simulink model "Grua_MC_R2_Ciclo_Completo_SFC"  (R2025b)
settings: Solver=ode23t  StartTime=0.0  StopTime=640  MaxStep=T_s  RelTol=1e-4
InitFcn:
  | addpath(fileparts(get_param(bdroot,'FileName')),'-begin');
  | run(fullfile(fileparts(get_param(bdroot,'FileName')),'definir_buses_variadores.m'));
  | run(fullfile(fileparts(get_param(bdroot,'FileName')),'parametros_ganancias_cascada_29072026.m'));
  | run(fullfile(fileparts(get_param(bdroot,'FileName')),'configurar_modelo_final_hmi.m'));
  | run(fullfile(fileparts(get_param(bdroot,'FileName')),'configurar_parametros_variadores.m'));
  | Pvis.Ts_viz=.04;Pvis.enable=true;Pvis.keepFigureOnTerminate=true;Pvis.hmi.fastDiagnostic=false;
undefined symbols (not defined in the file or in its folder): b_cx, b_cy, b_hb, b_hEb, b_heq, b_t, b_tb, b_teq, b_tw, b_wu, g, H_c, HMI, i_h, i_t, J_heq, J_teq, K_cy, K_tw, k_wu, L_h0, l_hi, M_c_profile, M_s, M_t, MC_FF, nLevels0, omega_hmRATED, r_hd, r_td, slotBlock, T_hbMax, T_hEbMax, T_hmMax, T_s, T_s1, T_tbMax, T_tmMax, tau_hm, tau_tm, traj_duration, traj_x_start, traj_x_target, v_hmaxLoaded, v_hmaxUnloaded, x_tmax, x_tmin, Y_c0, Y_t0, Zbase
libraries: simulink x1, aerolibanimutils x1
(part 3 of 4)

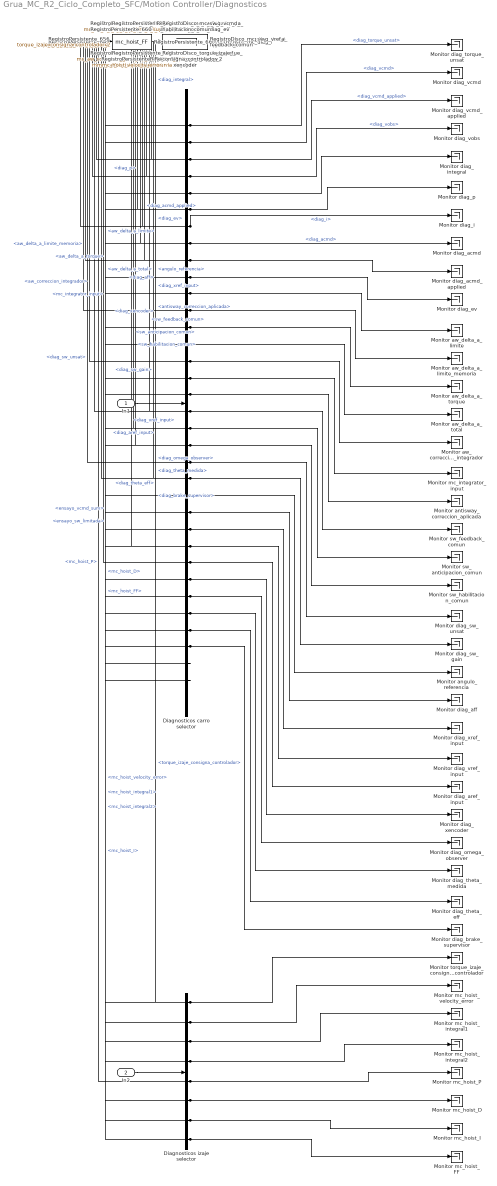
== system Grua_MC_R2_Ciclo_Completo_SFC/Motion Controller/Diagnosticos ==
  In1 : Inport
  In2 : Inport  Port=2
  Diagnosticos carro selector : BusSelector  OutputSignals=diag_torque_unsat,diag_vcmd,diag_vcmd_applied,diag_vobs,diag_integral,diag_p,diag_i,diag_acmd,diag_acmd_applied,diag_ev,aw_delta_a_limite,aw_delta_a_limite_memoria,aw_delta_a_torque,aw_delta_a_total,aw_correccion_integrador,mc_integrator_input,antisway_correccion_aplicada,sw_feedback_comun,sw_anticipacion_comun,sw_habilitacion_comun,diag_sw_unsat,diag_sw_gain,angulo_referencia,diag_aff,diag_xref_input,diag_vref_input,diag_aref_input,diag_xencoder,diag_omega_observer,diag_theta_medida,diag_theta_eff,diag_brake_supervisor,ensayo_vcmd_sum,ensayo_sw_limitada
  Diagnosticos izaje selector : BusSelector  OutputSignals=torque_izaje_consigna_controlador,mc_hoist_velocity_error,mc_hoist_integral1,mc_hoist_integral2,mc_hoist_P,mc_hoist_D,mc_hoist_I,mc_hoist_FF
  Monitor angulo_referencia : Terminator
  Monitor antisway_correccion_aplicada : Terminator
  Monitor aw_correccion_integrador : Terminator
  Monitor aw_delta_a_limite : Terminator
  Monitor aw_delta_a_limite_memoria : Terminator
  Monitor aw_delta_a_torque : Terminator
  Monitor aw_delta_a_total : Terminator
  Monitor diag_acmd : Terminator
  Monitor diag_acmd_applied : Terminator
  Monitor diag_aff : Terminator
  Monitor diag_aref_input : Terminator
  Monitor diag_brake_supervisor : Terminator
  Monitor diag_ev : Terminator
  Monitor diag_i : Terminator
  Monitor diag_integral : Terminator
  Monitor diag_omega_observer : Terminator
  Monitor diag_p : Terminator
  Monitor diag_sw_gain : Terminator
  Monitor diag_sw_unsat : Terminator
  Monitor diag_theta_eff : Terminator
  Monitor diag_theta_medida : Terminator
  Monitor diag_torque_unsat : Terminator
  Monitor diag_vcmd : Terminator
  Monitor diag_vcmd_applied : Terminator
  Monitor diag_vobs : Terminator
  Monitor diag_vref_input : Terminator
  Monitor diag_xencoder : Terminator
  Monitor diag_xref_input : Terminator
  Monitor mc_hoist_D : Terminator
  Monitor mc_hoist_FF : Terminator
  Monitor mc_hoist_I : Terminator
  Monitor mc_hoist_P : Terminator
  Monitor mc_hoist_integral1 : Terminator
  Monitor mc_hoist_integral2 : Terminator
  Monitor mc_hoist_velocity_error : Terminator
  Monitor mc_integrator_input : Terminator
  Monitor sw_anticipacion_comun : Terminator
  Monitor sw_feedback_comun : Terminator
  Monitor sw_habilitacion_comun : Terminator
  Monitor torque_izaje_consigna_controlador : Terminator
  RegistroDisco_angulo_referencia : Terminator
  RegistroDisco_mc_antisway_correccion_aplicada : Terminator
  RegistroDisco_mc_diag_acmd : Terminator
  RegistroDisco_mc_diag_acmd_applied : Terminator
  RegistroDisco_mc_diag_aff : Terminator
  RegistroDisco_mc_diag_aref_input : Terminator
  RegistroDisco_mc_diag_brake_supervisor : Terminator
  RegistroDisco_mc_diag_ev : Terminator
  RegistroDisco_mc_diag_i : Terminator
  RegistroDisco_mc_diag_integral : Terminator
  RegistroDisco_mc_diag_omega_observer : Terminator
  RegistroDisco_mc_diag_p : Terminator
  RegistroDisco_mc_diag_sw_gain : Terminator
  RegistroDisco_mc_diag_theta_eff : Terminator
  RegistroDisco_mc_diag_theta_medida : Terminator
  RegistroDisco_mc_diag_torque_unsat : Terminator
  RegistroDisco_mc_diag_vcmd : Terminator
  RegistroDisco_mc_diag_vcmd_applied : Terminator
  RegistroDisco_mc_diag_vobs : Terminator
  RegistroDisco_mc_diag_vref_input : Terminator
  RegistroDisco_mc_diag_xencoder : Terminator
  RegistroDisco_mc_diag_xref_input : Terminator
  RegistroDisco_mc_sw_anticipacion_comun : Terminator
  RegistroDisco_mc_sw_feedback_comun : Terminator
  RegistroDisco_mc_sw_habilitacion_comun : Terminator
  RegistroDisco_torque_izaje_consigna_controlador_2 : Terminator
  RegistroPersistente_622 : ToWorkspace  VariableName=mc_diag_torque_unsat  SaveFormat=Timeseries  SampleTime=-1
      settings: Decimation=10
  RegistroPersistente_623 : ToWorkspace  VariableName=mc_diag_vcmd  SaveFormat=Timeseries  SampleTime=-1
      settings: Decimation=10
  RegistroPersistente_624 : ToWorkspace  VariableName=mc_diag_vcmd_applied  SaveFormat=Timeseries  SampleTime=-1
      settings: Decimation=10
  RegistroPersistente_625 : ToWorkspace  VariableName=mc_diag_vobs  SaveFormat=Timeseries  SampleTime=-1
      settings: Decimation=10
  RegistroPersistente_626 : ToWorkspace  VariableName=mc_diag_integral  SaveFormat=Timeseries  SampleTime=-1
      settings: Decimation=10
  RegistroPersistente_627 : ToWorkspace  VariableName=mc_diag_p  SaveFormat=Timeseries  SampleTime=-1
      settings: Decimation=10
  RegistroPersistente_628 : ToWorkspace  VariableName=mc_diag_i  SaveFormat=Timeseries  SampleTime=-1
      settings: Decimation=10
  RegistroPersistente_629 : ToWorkspace  VariableName=mc_diag_acmd  SaveFormat=Timeseries  SampleTime=-1
      settings: Decimation=10
  RegistroPersistente_630 : ToWorkspace  VariableName=mc_diag_acmd_applied  SaveFormat=Timeseries  SampleTime=-1
      settings: Decimation=10
  RegistroPersistente_631 : ToWorkspace  VariableName=mc_diag_ev  SaveFormat=Timeseries  SampleTime=-1
      settings: Decimation=10
  RegistroPersistente_632 : ToWorkspace  VariableName=mc_aw_delta_a_limite  SaveFormat=Timeseries  SampleTime=-1
      settings: Decimation=10
  RegistroPersistente_633 : ToWorkspace  VariableName=mc_aw_delta_a_limite_memoria  SaveFormat=Timeseries  SampleTime=-1
      settings: Decimation=10
  RegistroPersistente_634 : ToWorkspace  VariableName=mc_aw_delta_a_torque  SaveFormat=Timeseries  SampleTime=-1
      settings: Decimation=10
  RegistroPersistente_635 : ToWorkspace  VariableName=mc_aw_delta_a_total  SaveFormat=Timeseries  SampleTime=-1
      settings: Decimation=10
  RegistroPersistente_636 : ToWorkspace  VariableName=mc_aw_correccion_integrador  SaveFormat=Timeseries  SampleTime=-1
      settings: Decimation=10
  RegistroPersistente_637 : ToWorkspace  VariableName=mc_mc_integrator_input  SaveFormat=Timeseries  SampleTime=-1
      settings: Decimation=10
  RegistroPersistente_638 : ToWorkspace  VariableName=mc_antisway_correccion_aplicada  SaveFormat=Timeseries  SampleTime=-1
      settings: Decimation=10
  RegistroPersistente_639 : ToWorkspace  VariableName=mc_sw_feedback_comun  SaveFormat=Timeseries  SampleTime=-1
      settings: Decimation=10
  RegistroPersistente_640 : ToWorkspace  VariableName=mc_sw_anticipacion_comun  SaveFormat=Timeseries  SampleTime=-1
      settings: Decimation=10
  RegistroPersistente_641 : ToWorkspace  VariableName=mc_sw_habilitacion_comun  SaveFormat=Timeseries  SampleTime=-1
      settings: Decimation=10
  RegistroPersistente_642 : ToWorkspace  VariableName=antisway_calculada  SaveFormat=Timeseries  SampleTime=-1
      settings: Decimation=10
  RegistroPersistente_643 : ToWorkspace  VariableName=mc_diag_sw_gain  SaveFormat=Timeseries  SampleTime=-1
      settings: Decimation=10
  RegistroPersistente_644 : ToWorkspace  VariableName=angulo_referencia  SaveFormat=Timeseries  SampleTime=-1
      settings: Decimation=10
  RegistroPersistente_645 : ToWorkspace  VariableName=mc_diag_aff  SaveFormat=Timeseries  SampleTime=-1
      settings: Decimation=10
  RegistroPersistente_646 : ToWorkspace  VariableName=mc_diag_xref_input  SaveFormat=Timeseries  SampleTime=-1
      settings: Decimation=10
  RegistroPersistente_647 : ToWorkspace  VariableName=mc_diag_vref_input  SaveFormat=Timeseries  SampleTime=-1
      settings: Decimation=10
  RegistroPersistente_648 : ToWorkspace  VariableName=mc_diag_aref_input  SaveFormat=Timeseries  SampleTime=-1
      settings: Decimation=10
  RegistroPersistente_649 : ToWorkspace  VariableName=mc_diag_xencoder  SaveFormat=Timeseries  SampleTime=-1
      settings: Decimation=10
  RegistroPersistente_650 : ToWorkspace  VariableName=mc_diag_omega_observer  SaveFormat=Timeseries  SampleTime=-1
      settings: Decimation=10
  RegistroPersistente_651 : ToWorkspace  VariableName=mc_diag_theta_medida  SaveFormat=Timeseries  SampleTime=-1
      settings: Decimation=10
  RegistroPersistente_652 : ToWorkspace  VariableName=mc_diag_theta_eff  SaveFormat=Timeseries  SampleTime=-1
      settings: Decimation=10
  RegistroPersistente_653 : ToWorkspace  VariableName=mc_diag_brake_supervisor  SaveFormat=Timeseries  SampleTime=-1
      settings: Decimation=10
  RegistroPersistente_654 : ToWorkspace  VariableName=v_cmd  SaveFormat=Timeseries  SampleTime=-1
      settings: Decimation=10
  RegistroPersistente_655 : ToWorkspace  VariableName=antisway_limitada  SaveFormat=Timeseries  SampleTime=-1
      settings: Decimation=10
  RegistroPersistente_656 : ToWorkspace  VariableName=torque_izaje_consigna_controlador_2  SaveFormat=Timeseries  SampleTime=-1
      settings: Decimation=10
  RegistroPersistente_657 : ToWorkspace  VariableName=mc_hoist_velocity_error  SaveFormat=Timeseries  SampleTime=-1
      settings: Decimation=10
  RegistroPersistente_658 : ToWorkspace  VariableName=mc_hoist_integral1  SaveFormat=Timeseries  SampleTime=-1
      settings: Decimation=10
  RegistroPersistente_659 : ToWorkspace  VariableName=mc_hoist_integral2  SaveFormat=Timeseries  SampleTime=-1
      settings: Decimation=10
  RegistroPersistente_660 : ToWorkspace  VariableName=mc_hoist_P  SaveFormat=Timeseries  SampleTime=-1
      settings: Decimation=10
  RegistroPersistente_661 : ToWorkspace  VariableName=mc_hoist_D  SaveFormat=Timeseries  SampleTime=-1
      settings: Decimation=10
  RegistroPersistente_662 : ToWorkspace  VariableName=mc_hoist_I  SaveFormat=Timeseries  SampleTime=-1
      settings: Decimation=10
  RegistroPersistente_663 : ToWorkspace  VariableName=mc_hoist_FF  SaveFormat=Timeseries  SampleTime=-1
      settings: Decimation=10
  wires:
  Diagnosticos izaje selector/6 -> Monitor mc_hoist_D/1, RegistroPersistente_661/1  "<mc_hoist_D>"
  Diagnosticos carro selector/27 -> Monitor diag_aref_input/1, RegistroPersistente_648/1, RegistroDisco_mc_diag_aref_input/1  "<diag_aref_input>"
  In1/1 -> Diagnosticos carro selector/1
  Diagnosticos carro selector/22 -> Monitor diag_sw_gain/1, RegistroPersistente_643/1, RegistroDisco_mc_diag_sw_gain/1  "<diag_sw_gain>"
  Diagnosticos izaje selector/5 -> Monitor mc_hoist_P/1, RegistroPersistente_660/1  "<mc_hoist_P>"
  Diagnosticos carro selector/3 -> Monitor diag_vcmd_applied/1, RegistroPersistente_624/1, RegistroDisco_mc_diag_vcmd_applied/1  "<diag_vcmd_applied>"
  Diagnosticos carro selector/18 -> Monitor sw_feedback_comun/1, RegistroPersistente_639/1, RegistroDisco_mc_sw_feedback_comun/1  "<sw_feedback_comun>"
  Diagnosticos carro selector/4 -> Monitor diag_vobs/1, RegistroPersistente_625/1, RegistroDisco_mc_diag_vobs/1  "<diag_vobs>"
  Diagnosticos carro selector/15 -> Monitor aw_correccion_integrador/1, RegistroPersistente_636/1  "<aw_correccion_integrador>"
  In2/1 -> Diagnosticos izaje selector/1
  Diagnosticos carro selector/21 -> Monitor diag_sw_unsat/1, RegistroPersistente_642/1  "<diag_sw_unsat>"
  Diagnosticos carro selector/9 -> Monitor diag_acmd_applied/1, RegistroPersistente_630/1, RegistroDisco_mc_diag_acmd_applied/1  "<diag_acmd_applied>"
  Diagnosticos carro selector/12 -> Monitor aw_delta_a_limite_memoria/1, RegistroPersistente_633/1  "<aw_delta_a_limite_memoria>"
  Diagnosticos carro selector/7 -> Monitor diag_i/1, RegistroPersistente_628/1, RegistroDisco_mc_diag_i/1  "<diag_i>"
  Diagnosticos carro selector/8 -> Monitor diag_acmd/1, RegistroPersistente_629/1, RegistroDisco_mc_diag_acmd/1  "<diag_acmd>"
  Diagnosticos carro selector/6 -> Monitor diag_p/1, RegistroPersistente_627/1, RegistroDisco_mc_diag_p/1  "<diag_p>"
  Diagnosticos carro selector/20 -> Monitor sw_habilitacion_comun/1, RegistroPersistente_641/1, RegistroDisco_mc_sw_habilitacion_comun/1  "<sw_habilitacion_comun>"
  Diagnosticos carro selector/19 -> Monitor sw_anticipacion_comun/1, RegistroPersistente_640/1, RegistroDisco_mc_sw_anticipacion_comun/1  "<sw_anticipacion_comun>"
  Diagnosticos carro selector/26 -> Monitor diag_vref_input/1, RegistroPersistente_647/1, RegistroDisco_mc_diag_vref_input/1  "<diag_vref_input>"
  Diagnosticos carro selector/11 -> Monitor aw_delta_a_limite/1, RegistroPersistente_632/1  "<aw_delta_a_limite>"
  Diagnosticos carro selector/32 -> Monitor diag_brake_supervisor/1, RegistroPersistente_653/1, RegistroDisco_mc_diag_brake_supervisor/1  "<diag_brake_supervisor>"
  Diagnosticos carro selector/13 -> Monitor aw_delta_a_torque/1, RegistroPersistente_634/1  "<aw_delta_a_torque>"
  Diagnosticos carro selector/2 -> Monitor diag_vcmd/1, RegistroPersistente_623/1, RegistroDisco_mc_diag_vcmd/1  "<diag_vcmd>"
  Diagnosticos carro selector/17 -> Monitor antisway_correccion_aplicada/1, RegistroPersistente_638/1, RegistroDisco_mc_antisway_correccion_aplicada/1  "<antisway_correccion_aplicada>"
  Diagnosticos izaje selector/1 -> Monitor torque_izaje_consigna_controlador/1, RegistroPersistente_656/1, RegistroDisco_torque_izaje_consigna_controlador_2/1  "<torque_izaje_consigna_controlador>"
  Diagnosticos carro selector/10 -> Monitor diag_ev/1, RegistroPersistente_631/1, RegistroDisco_mc_diag_ev/1  "<diag_ev>"
  Diagnosticos carro selector/1 -> Monitor diag_torque_unsat/1, RegistroPersistente_622/1, RegistroDisco_mc_diag_torque_unsat/1  "<diag_torque_unsat>"
  Diagnosticos carro selector/5 -> Monitor diag_integral/1, RegistroPersistente_626/1, RegistroDisco_mc_diag_integral/1  "<diag_integral>"
  Diagnosticos carro selector/16 -> Monitor mc_integrator_input/1, RegistroPersistente_637/1  "<mc_integrator_input>"
  Diagnosticos izaje selector/4 -> Monitor mc_hoist_integral2/1, RegistroPersistente_659/1  "<mc_hoist_integral2>"
  Diagnosticos izaje selector/2 -> Monitor mc_hoist_velocity_error/1, RegistroPersistente_657/1  "<mc_hoist_velocity_error>"
  Diagnosticos izaje selector/3 -> Monitor mc_hoist_integral1/1, RegistroPersistente_658/1  "<mc_hoist_integral1>"
  Diagnosticos carro selector/14 -> Monitor aw_delta_a_total/1, RegistroPersistente_635/1  "<aw_delta_a_total>"
  Diagnosticos carro selector/28 -> Monitor diag_xencoder/1, RegistroPersistente_649/1, RegistroDisco_mc_diag_xencoder/1  "<diag_xencoder>"
  Diagnosticos carro selector/24 -> Monitor diag_aff/1, RegistroPersistente_645/1, RegistroDisco_mc_diag_aff/1  "<diag_aff>"
  Diagnosticos carro selector/23 -> Monitor angulo_referencia/1, RegistroPersistente_644/1, RegistroDisco_angulo_referencia/1  "<angulo_referencia>"
  Diagnosticos carro selector/30 -> Monitor diag_theta_medida/1, RegistroPersistente_651/1, RegistroDisco_mc_diag_theta_medida/1  "<diag_theta_medida>"
  Diagnosticos carro selector/31 -> Monitor diag_theta_eff/1, RegistroPersistente_652/1, RegistroDisco_mc_diag_theta_eff/1  "<diag_theta_eff>"
  Diagnosticos carro selector/29 -> Monitor diag_omega_observer/1, RegistroPersistente_650/1, RegistroDisco_mc_diag_omega_observer/1  "<diag_omega_observer>"
  Diagnosticos carro selector/25 -> Monitor diag_xref_input/1, RegistroPersistente_646/1, RegistroDisco_mc_diag_xref_input/1  "<diag_xref_input>"
  Diagnosticos izaje selector/8 -> Monitor mc_hoist_FF/1, RegistroPersistente_663/1  "<mc_hoist_FF>"
  Diagnosticos izaje selector/7 -> Monitor mc_hoist_I/1, RegistroPersistente_662/1  "<mc_hoist_I>"
  Diagnosticos carro selector/33 -> RegistroPersistente_654/1  "<ensayo_vcmd_sum>"
  Diagnosticos carro selector/34 -> RegistroPersistente_655/1  "<ensayo_sw_limitada>"

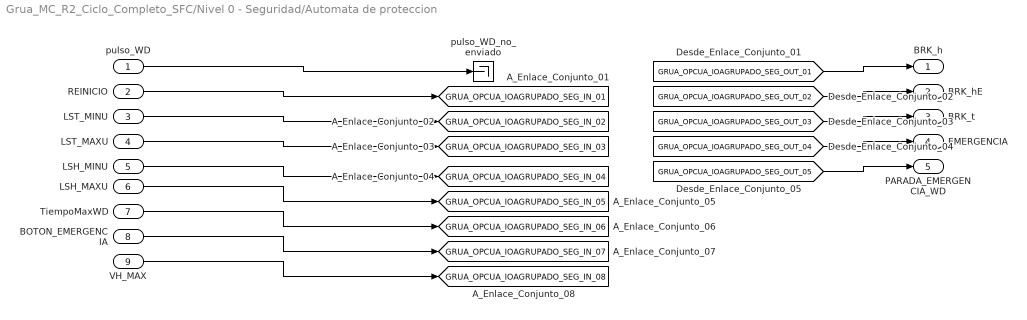
== system Grua_MC_R2_Ciclo_Completo_SFC/Nivel 0 - Seguridad/Automata de proteccion ==
  pulso_WD : Inport
  REINICIO : Inport  Port=2
  LST_MINU : Inport  Port=3
  LST_MAXU : Inport  Port=4
  LSH_MINU : Inport  Port=5
  LSH_MAXU : Inport  Port=6
  TiempoMaxWD : Inport  Port=7
  BOTON_EMERGENCIA : Inport  Port=8
  VH_MAX : Inport  Port=9
  pulso_WD_no_enviado : Terminator
  BRK_h : Outport
  BRK_hE : Outport  Port=2
  BRK_t : Outport  Port=3
  EMERGENCIA : Outport  Port=4
  PARADA_EMERGENCIA_WD : Outport  Port=5
  tag scope: GRUA_OPCUA_IOAGRUPADO_SEG_IN_01=global, GRUA_OPCUA_IOAGRUPADO_SEG_IN_02=global, GRUA_OPCUA_IOAGRUPADO_SEG_IN_03=global, GRUA_OPCUA_IOAGRUPADO_SEG_IN_04=global, GRUA_OPCUA_IOAGRUPADO_SEG_IN_05=global, GRUA_OPCUA_IOAGRUPADO_SEG_IN_06=global, GRUA_OPCUA_IOAGRUPADO_SEG_IN_07=global, GRUA_OPCUA_IOAGRUPADO_SEG_IN_08=global
  wires:
  [GRUA_OPCUA_IOAGRUPADO_SEG_OUT_05] -> PARADA_EMERGENCIA_WD/1
  [GRUA_OPCUA_IOAGRUPADO_SEG_OUT_04] -> EMERGENCIA/1
  [GRUA_OPCUA_IOAGRUPADO_SEG_OUT_03] -> BRK_t/1
  [GRUA_OPCUA_IOAGRUPADO_SEG_OUT_02] -> BRK_hE/1
  [GRUA_OPCUA_IOAGRUPADO_SEG_OUT_01] -> BRK_h/1
  VH_MAX/1 -> [GRUA_OPCUA_IOAGRUPADO_SEG_IN_08]
  BOTON_EMERGENCIA/1 -> [GRUA_OPCUA_IOAGRUPADO_SEG_IN_07]
  TiempoMaxWD/1 -> [GRUA_OPCUA_IOAGRUPADO_SEG_IN_06]
  LSH_MAXU/1 -> [GRUA_OPCUA_IOAGRUPADO_SEG_IN_05]
  LSH_MINU/1 -> [GRUA_OPCUA_IOAGRUPADO_SEG_IN_04]
  LST_MAXU/1 -> [GRUA_OPCUA_IOAGRUPADO_SEG_IN_03]
  LST_MINU/1 -> [GRUA_OPCUA_IOAGRUPADO_SEG_IN_02]
  REINICIO/1 -> [GRUA_OPCUA_IOAGRUPADO_SEG_IN_01]
  pulso_WD/1 -> pulso_WD_no_enviado/1

== system Grua_MC_R2_Ciclo_Completo_SFC/Planta/Calculo longitud l ==
  x_l : Inport
  y_l : Inport  Port=2
  v_lx : Inport  Port=3
  v_ly : Inport  Port=4
  x_t : Inport  Port=5
  v_t : Inport  Port=6
  Constant : Constant  Value=Y_t0
  Divide : Product  Inputs=*/
  Product : Product
  Product1 : Product
  Sqrt : Sqrt
  Square : Math  Operator=square
  Square1 : Math  Operator=square
  Sum : Sum  Inputs=|+-
  Sum1 : Sum  Inputs=|+-
  Sum2 : Sum
  Sum3 : Sum  Inputs=|+-
  Sum4 : Sum  Inputs=+-
  l : Outport
  dl : Outport  Port=2
  wires:
  Sqrt/1 -> Divide/2, l/1  "l"
  x_l/1 -> Sum/1
  x_t/1 -> Sum/2
  Sum/1 -> Product/1, Square/1
  Constant/1 -> Sum1/1
  y_l/1 -> Sum1/2
  Sum1/1 -> Product1/1, Square1/1
  Square1/1 -> Sum2/2
  Square/1 -> Sum2/1
  Sum2/1 -> Sqrt/1
  v_lx/1 -> Sum3/1
  v_t/1 -> Sum3/2
  Sum3/1 -> Product/2
  v_ly/1 -> Product1/2
  Product1/1 -> Sum4/2
  Product/1 -> Sum4/1
  Sum4/1 -> Divide/1
  Divide/1 -> dl/1  "dl"

== system Grua_MC_R2_Ciclo_Completo_SFC/Planta/Subsistema carga ==
  x_t : Inport
  F_w : Inport  Port=2
  M_c : Inport  Port=3
  y_c0(x_l,t) : Inport  Port=4
  TLK : Inport  Port=5
  Calculo Angulo De Balanceo : Subsystem
  Calculo Fuerza De Contacto : Subsystem
  Calculo Longitud Inferior : Subsystem
  Calculo Masa Total de Carga : Subsystem
  Derivative : Derivative
  Dinamica Movimiento Carga : Subsystem
  RegistroDisco_masa_fisica_suspendida : Terminator
  RegistroDisco_v_izaje_fisica : Terminator
  RegistroDisco_y_carga_fisica : Terminator
  RegistroPersistente_830 : ToWorkspace  VariableName=masa_fisica_suspendida  SaveFormat=Timeseries  SampleTime=-1
      settings: Decimation=10
  RegistroPersistente_838 : ToWorkspace  VariableName=y_carga_fisica  SaveFormat=Timeseries  SampleTime=-1
      settings: Decimation=10
  RegistroPersistente_840 : ToWorkspace  VariableName=v_izaje_fisica  SaveFormat=Timeseries  SampleTime=-1
      settings: Decimation=10
  x_l : Outport
  y_l : Outport  Port=2
  v_lx : Outport  Port=3
  v_ly : Outport  Port=4
  theta_l : Outport  Port=5
  omega_l : Outport  Port=6
  F_cy : Outport  Port=7
  wires:
  Calculo Fuerza De Contacto/2(F_cy) -> F_cy/1, Dinamica Movimiento Carga/3(F_cy)
  Dinamica Movimiento Carga/4(v_ly) -> v_ly/1, Calculo Fuerza De Contacto/3(v_ly), RegistroPersistente_840/1, RegistroDisco_v_izaje_fisica/1
  x_t/1 -> Calculo Angulo De Balanceo/3(x_t)
  Dinamica Movimiento Carga/2(y_l) -> y_l/1, Calculo Angulo De Balanceo/2(y_l), Calculo Fuerza De Contacto/1(y_l), RegistroPersistente_838/1, RegistroDisco_y_carga_fisica/1
  Calculo Angulo De Balanceo/1(theta_l) -> Dinamica Movimiento Carga/5(theta_l), Derivative/1, theta_l/1
  y_c0(x_l,t)/1 -> Calculo Fuerza De Contacto/5(y_c0(x_l,t))
  Calculo Fuerza De Contacto/1(F_cx) -> Dinamica Movimiento Carga/2(F_cx)
  Dinamica Movimiento Carga/1(x_l) -> x_l/1, Calculo Angulo De Balanceo/1(x_l)
  Dinamica Movimiento Carga/3(v_lx) -> v_lx/1, Calculo Fuerza De Contacto/2(v_lx)
  Calculo Longitud Inferior/1(h_c) -> Calculo Fuerza De Contacto/4(h_c)
  F_w/1 -> Dinamica Movimiento Carga/4(F_hw)
  M_c/1 -> Calculo Masa Total de Carga/2(M_c)
  TLK/1 -> Calculo Longitud Inferior/1(TLK), Calculo Masa Total de Carga/1(TLK)
  Derivative/1 -> omega_l/1
  Calculo Masa Total de Carga/1(m_l) -> Dinamica Movimiento Carga/1(m_l), RegistroPersistente_830/1, RegistroDisco_masa_fisica_suspendida/1

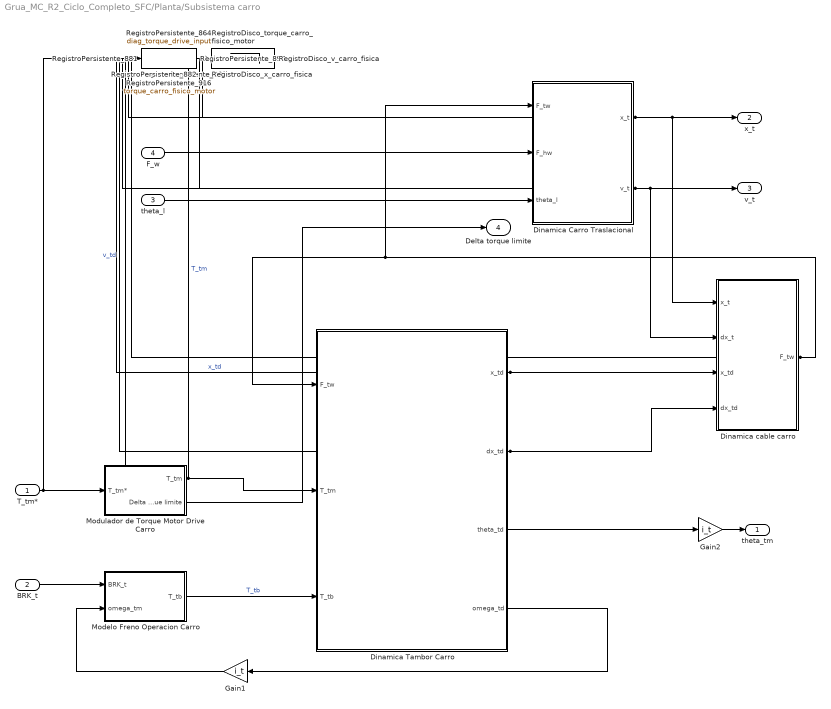
== system Grua_MC_R2_Ciclo_Completo_SFC/Planta/Subsistema carro ==
  T_tm* : Inport
  BRK_t : Inport  Port=2
  theta_l : Inport  Port=3
  F_w : Inport  Port=4
  Dinamica Carro Traslacional : Subsystem
  Dinamica Tambor Carro : Subsystem
  Dinamica cable carro : Subsystem
  Gain1 : Gain  Gain=i_t
  Gain2 : Gain  Gain=i_t
  Modelo Freno Operacion Carro : Subsystem
  Modulador de Torque Motor Drive Carro : Subsystem
  RegistroDisco_torque_carro_fisico_motor : Terminator
  RegistroDisco_v_carro_fisica : Terminator
  RegistroDisco_x_carro_fisica : Terminator
  RegistroPersistente_864 : ToWorkspace  VariableName=diag_torque_drive_input  SaveFormat=Timeseries  SampleTime=-1
      settings: Decimation=10
  RegistroPersistente_868 : ToWorkspace  VariableName=x_carro_fisica  SaveFormat=Timeseries  SampleTime=-1
      settings: Decimation=10
  RegistroPersistente_869 : ToWorkspace  VariableName=v_carro_fisica  SaveFormat=Timeseries  SampleTime=-1
      settings: Decimation=10
  RegistroPersistente_881 : ToWorkspace  VariableName=x_td  SaveFormat=Timeseries  SampleTime=-1
      settings: Decimation=10
  RegistroPersistente_882 : ToWorkspace  VariableName=v_td  SaveFormat=Timeseries  SampleTime=-1
      settings: Decimation=10
  RegistroPersistente_897 : ToWorkspace  VariableName=diag_traction  SaveFormat=Timeseries  SampleTime=-1
      settings: Decimation=10
  RegistroPersistente_916 : ToWorkspace  VariableName=torque_carro_fisico_motor  SaveFormat=Timeseries  SampleTime=-1
      settings: Decimation=10
  theta_tm : Outport
  x_t : Outport  Port=2
  v_t : Outport  Port=3
  Delta torque limite : Outport  Port=4
  wires:
  Dinamica cable carro/1(F_tw) -> Dinamica Carro Traslacional/1(F_tw), Dinamica Tambor Carro/1(F_tw), RegistroPersistente_897/1
  Gain1/1 -> Modelo Freno Operacion Carro/2(omega_tm)
  F_w/1 -> Dinamica Carro Traslacional/2(F_hw)
  Dinamica Carro Traslacional/1(x_t) -> x_t/1, Dinamica cable carro/1(x_t), RegistroPersistente_868/1, RegistroDisco_x_carro_fisica/1
  Modulador de Torque Motor Drive Carro/1(T_tm) -> Dinamica Tambor Carro/2(T_tm), RegistroPersistente_916/1, RegistroDisco_torque_carro_fisico_motor/1  "T_tm"
  Dinamica Tambor Carro/4(omega_td) -> Gain1/1
  Dinamica Carro Traslacional/2(v_t) -> v_t/1, Dinamica cable carro/2(dx_t), RegistroPersistente_869/1, RegistroDisco_v_carro_fisica/1
  Dinamica Tambor Carro/2(dx_td) -> Dinamica cable carro/4(dx_td), RegistroPersistente_882/1  "v_td"
  Dinamica Tambor Carro/1(x_td) -> Dinamica cable carro/3(x_td), RegistroPersistente_881/1  "x_td"
  Modelo Freno Operacion Carro/1(T_tb) -> Dinamica Tambor Carro/3(T_tb)  "T_tb"
  BRK_t/1 -> Modelo Freno Operacion Carro/1(BRK_t)
  Dinamica Tambor Carro/3(theta_td) -> Gain2/1
  T_tm*/1 -> Modulador de Torque Motor Drive Carro/1(T_tm*), RegistroPersistente_864/1
  theta_l/1 -> Dinamica Carro Traslacional/3(theta_l)
  Gain2/1 -> theta_tm/1
  Modulador de Torque Motor Drive Carro/2(Delta torque limite) -> Delta torque limite/1

== system Grua_MC_R2_Ciclo_Completo_SFC/Planta/Subsistema izaje ==
  F_hw : Inport
  BRK_hE : Inport  Port=2
  T_hm* : Inport  Port=3
  BRK_h : Inport  Port=4
  l : Inport  Port=5
  dl : Inport  Port=6
  Calculo longitud l_h : Subsystem
  Dinamica Tambor Izaje : Subsystem
  Dinamica cable Izaje : Subsystem
  Gain : Gain  Gain=i_h
  Gain1 : Gain  Gain=i_h
  Modelo Freno Emergencia de Izaje(Eje lento) : Subsystem
  Modelo Freno Operacion de Izaje(Eje Rapido) : Subsystem
  Modulador de Torque Motor Drive Izaje : Subsystem
  RegistroDisco_torque_izaje_fisico_motor : Terminator
  RegistroPersistente_934 : ToWorkspace  VariableName=l_h  SaveFormat=Timeseries  SampleTime=-1
      settings: Decimation=10
  RegistroPersistente_992 : ToWorkspace  VariableName=torque_izaje_fisico_motor  SaveFormat=Timeseries  SampleTime=-1
      settings: Decimation=10
  theta_hd : Outport
  theta_hm : Outport  Port=2
  F_w : Outport  Port=3
  omega_hd : Outport  Port=4
  wires:
  Calculo longitud l_h/1(l_h) -> Dinamica cable Izaje/2(l_h), RegistroPersistente_934/1  "l_h"
  Calculo longitud l_h/2(dl_h) -> Dinamica cable Izaje/4(dl_h)
  F_hw/1 -> Dinamica Tambor Izaje/3(F_hw)
  Modelo Freno Emergencia de Izaje(Eje lento)/1(T_hEb) -> Dinamica Tambor Izaje/1(T_hEb)
  Dinamica Tambor Izaje/1(theta_hd) -> Gain1/1, theta_hd/1
  BRK_h/1 -> Modelo Freno Operacion de Izaje(Eje Rapido)/1(BRK_h)
  Modelo Freno Operacion de Izaje(Eje Rapido)/1(T_hb) -> Dinamica Tambor Izaje/4(T_hb)
  Gain/1 -> Modulador de Torque Motor Drive Izaje/2(omega_hm), Modelo Freno Operacion de Izaje(Eje Rapido)/2(omega_hm)
  BRK_hE/1 -> Modelo Freno Emergencia de Izaje(Eje lento)/2(BRK_hE)
  T_hm*/1 -> Modulador de Torque Motor Drive Izaje/1(T_hm*)
  l/1 -> Dinamica cable Izaje/1(l)
  Dinamica cable Izaje/1(F_hw) -> F_w/1  "F_w"
  dl/1 -> Dinamica cable Izaje/3(dl)
  Modulador de Torque Motor Drive Izaje/1(T_hm) -> Dinamica Tambor Izaje/2(T_hm), RegistroPersistente_992/1, RegistroDisco_torque_izaje_fisico_motor/1
  Gain1/1 -> theta_hm/1
  Dinamica Tambor Izaje/2(omega_hd) -> Gain/1, Modelo Freno Emergencia de Izaje(Eje lento)/1(omega_hd), Calculo longitud l_h/1(omega_hd), omega_hd/1

== system Grua_MC_R2_Ciclo_Completo_SFC/SENSORES/Finales de carrera operacion carro ==
  x_t : Inport
  Constant : Constant  Value=x_tmax
  Constant1 : Constant  Value=x_tmin
  Constant2 : Constant  Value=x_tmax+0.50
  Constant3 : Constant  Value=x_tmin-0.50
  Relational Operator{1..4} (4 alike) : RelationalOperator  OutDataTypeStr=boolean  RndMeth=Simplest  InputSameDT=off
  x_tLSmax : Outport
  x_tLSmin : Outport  Port=2
  x_tLSEmax : Outport  Port=3
  x_tLSEmin : Outport  Port=4
  wires:
  Relational Operator4/1 -> x_tLSmax/1
  Constant/1 -> Relational Operator4/2
  Constant1/1 -> Relational Operator1/1
  x_t/1 -> Relational Operator3/2, Relational Operator2/1, Relational Operator1/2, Relational Operator4/1
  Relational Operator1/1 -> x_tLSmin/1
  Relational Operator3/1 -> x_tLSEmin/1
  Relational Operator2/1 -> x_tLSEmax/1
  Constant2/1 -> Relational Operator2/2
  Constant3/1 -> Relational Operator3/1

== system Grua_MC_R2_Ciclo_Completo_SFC/SENSORES/Sensor de Sobrevelocidad>115% ==
  v_h : Inport
  TLK : Inport  Port=2
  Abs : Abs  SaturateOnIntegerOverflow=off
  Constant : Constant  Value=v_hmaxLoaded
  Constant1 : Constant  Value=v_hmaxUnloaded
  Gain : Gain  Gain=1.15
  Relational Operator : RelationalOperator  OutDataTypeStr=boolean  RndMeth=Simplest  InputSameDT=off
  Switch : Switch  Criteria=u2 > Threshold  SaturateOnIntegerOverflow=off  InputSameDT=off
  Sobrevelocidad : Outport
  wires:
  Switch/1 -> Gain/1  "v_hlim"
  Constant/1 -> Switch/1
  TLK/1 -> Switch/2
  Constant1/1 -> Switch/3
  v_h/1 -> Abs/1
  Relational Operator/1 -> Sobrevelocidad/1
  Gain/1 -> Relational Operator/2
  Abs/1 -> Relational Operator/1

== system Grua_MC_R2_Ciclo_Completo_SFC/SENSORES/Subsystem1 ==
  theta_l : Inport
  omega_l : Inport  Port=2
  sensor angulo vertical : Gain
  sensor de velocidad angular : Gain
  theta_l_sensor : Outport
  omega_l_sensor : Outport  Port=2
  wires:
  sensor angulo vertical/1 -> theta_l_sensor/1
  sensor de velocidad angular/1 -> omega_l_sensor/1
  omega_l/1 -> sensor de velocidad angular/1
  theta_l/1 -> sensor angulo vertical/1

== system Grua_MC_R2_Ciclo_Completo_SFC/Planta/Subsistema carga/Calculo Angulo De Balanceo ==
  x_l : Inport
  y_l : Inport  Port=2
  x_t : Inport  Port=3
  Atan : Trigonometry  Operator=atan2
  Constant : Constant  Value=Y_t0
  RegistroPersistente_802 : ToWorkspace  VariableName=x_l  SaveFormat=Timeseries  SampleTime=-1
      settings: Decimation=10
  RegistroPersistente_803 : ToWorkspace  VariableName=y_l  SaveFormat=Timeseries  SampleTime=-1
      settings: Decimation=10
  RegistroPersistente_804 : ToWorkspace  VariableName=x_t  SaveFormat=Timeseries  SampleTime=-1
      settings: Decimation=10
  Sum : Sum  Inputs=|+-
  Sum1 : Sum  Inputs=|+-
  theta_l : Outport
  wires:
  x_l/1 -> Sum/1, RegistroPersistente_802/1  "x_l"
  x_t/1 -> Sum/2, RegistroPersistente_804/1  "x_t"
  Constant/1 -> Sum1/1
  y_l/1 -> Sum1/2, RegistroPersistente_803/1  "y_l"
  Sum/1 -> Atan/1
  Sum1/1 -> Atan/2
  Atan/1 -> theta_l/1

== system Grua_MC_R2_Ciclo_Completo_SFC/Planta/Subsistema carga/Calculo Fuerza De Contacto ==
  y_l : Inport
  v_lx : Inport  Port=2
  v_ly : Inport  Port=3
  h_c : Inport  Port=4
  y_c0(x_l,t) : Inport  Port=5
  Constant1 : Constant  Value=0
  Gain : Gain  Gain=-b_cx
  Gain1 : Gain  Gain=K_cy
  Gain2 : Gain  Gain=-b_cy
  Limite fuerza contacto : Saturate  UpperLimit=2e6  LowerLimit=0
  RegistroPersistente_821 : ToWorkspace  VariableName=sumFcx  SaveFormat=Timeseries  SampleTime=-1
      settings: Decimation=10
  RegistroPersistente_823 : ToWorkspace  VariableName=registro_823  SaveFormat=Timeseries  SampleTime=-1
      settings: Decimation=10
  Sum : Sum  Inputs=++-
  Sum1 : Sum  Inputs=|++
  Switch : Switch  SaturateOnIntegerOverflow=off  InputSameDT=off
  Switch1 : Switch  SaturateOnIntegerOverflow=off  InputSameDT=off
  F_cx : Outport
  F_cy : Outport  Port=2
  wires:
  Switch/1 -> F_cx/1, RegistroPersistente_823/1
  Constant1/1 -> Switch1/3, Switch/3
  Gain/1 -> Switch/1
  h_c/1 -> Sum/2
  y_c0(x_l,t)/1 -> Sum/1
  y_l/1 -> Sum/3
  Sum/1 -> Gain1/1, Switch1/2, Switch/2, RegistroPersistente_821/1  "sumFcx"
  v_lx/1 -> Gain/1
  Gain1/1 -> Sum1/1
  Gain2/1 -> Sum1/2
  v_ly/1 -> Gain2/1
  Sum1/1 -> Switch1/1
  Switch1/1 -> Limite fuerza contacto/1
  Limite fuerza contacto/1 -> F_cy/1

== system Grua_MC_R2_Ciclo_Completo_SFC/Planta/Subsistema carga/Calculo Longitud Inferior ==
  TLK : Inport
  Constant : Constant  Value=H_c
  Constant1 : Constant  Value=0
  Switch : Switch  Criteria=u2 > Threshold  SaturateOnIntegerOverflow=off  InputSameDT=off
  h_c : Outport
  wires:
  TLK/1 -> Switch/2
  Switch/1 -> h_c/1
  Constant1/1 -> Switch/3
  Constant/1 -> Switch/1

== system Grua_MC_R2_Ciclo_Completo_SFC/Planta/Subsistema carga/Calculo Masa Total de Carga ==
  TLK : Inport
  M_c : Inport  Port=2
  Constant : Constant  Value=M_s
  Sum : Sum  Inputs=|++
  Switch : Switch  Criteria=u2 > Threshold  SaturateOnIntegerOverflow=off  InputSameDT=off
  m_l : Outport
  wires:
  TLK/1 -> Switch/2
  M_c/1 -> Sum/2
  Switch/1 -> m_l/1
  Constant/1 -> Sum/1, Switch/3
  Sum/1 -> Switch/1

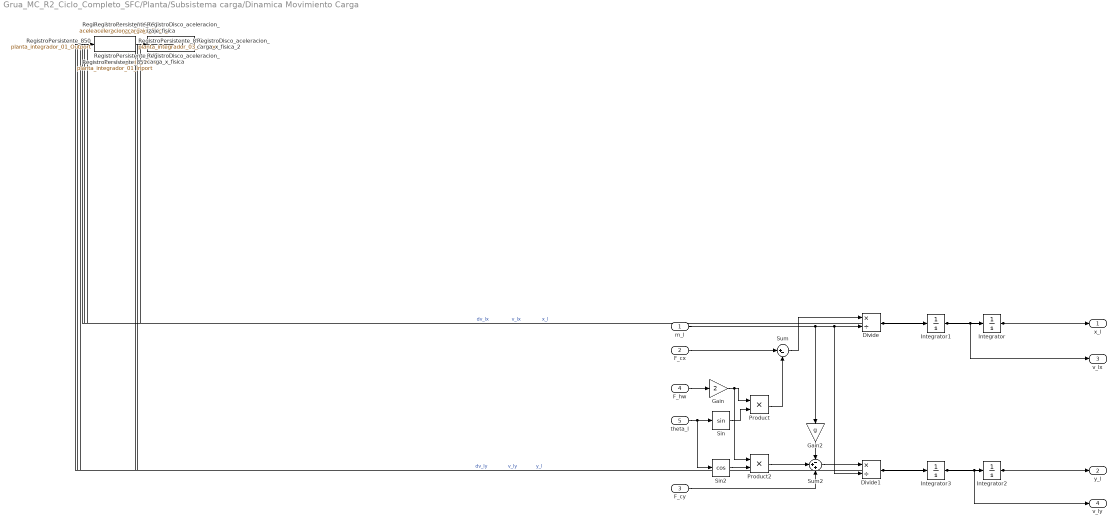
== system Grua_MC_R2_Ciclo_Completo_SFC/Planta/Subsistema carga/Dinamica Movimiento Carga ==
  m_l : Inport
  F_cx : Inport  Port=2
  F_cy : Inport  Port=3
  F_hw : Inport  Port=4
  theta_l : Inport  Port=5
  Divide : Product  Inputs=*/
  Divide1 : Product  Inputs=*/
  Gain : Gain  Gain=2
  Gain2 : Gain  Gain=g
  Integrator : Integrator  InitialCondition=-26.34
  Integrator1 : Integrator
  Integrator2 : Integrator  InitialCondition=25
  Integrator3 : Integrator
  Product : Product
  Product2 : Product
  RegistroDisco_aceleracion_carga_x_fisica : Terminator
  RegistroDisco_aceleracion_carga_x_fisica_2 : Terminator
  RegistroDisco_aceleracion_izaje_fisica : Terminator
  RegistroPersistente_846 : ToWorkspace  VariableName=aceleracion_carga_x_fisica  SaveFormat=Timeseries  SampleTime=-1
      settings: Decimation=10
  RegistroPersistente_847 : ToWorkspace  VariableName=aceleracion_izaje_fisica  SaveFormat=Timeseries  SampleTime=-1
      settings: Decimation=10
  RegistroPersistente_850 : ToWorkspace  VariableName=planta_integrador_01_Outport  SaveFormat=Timeseries  SampleTime=-1
      settings: Decimation=10
  RegistroPersistente_851 : ToWorkspace  VariableName=planta_integrador_01_Inport  SaveFormat=Timeseries  SampleTime=-1
      settings: Decimation=10
  RegistroPersistente_852 : ToWorkspace  VariableName=planta_integrador_03_Outport  SaveFormat=Timeseries  SampleTime=-1
      settings: Decimation=10
  RegistroPersistente_853 : ToWorkspace  VariableName=aceleracion_carga_x_fisica_2  SaveFormat=Timeseries  SampleTime=-1
      settings: Decimation=10
  Sin : Trigonometry
  Sin2 : Trigonometry  Operator=cos
  Sum : Sum  Inputs=|+-
  Sum2 : Sum  Inputs=-++
  x_l : Outport
  y_l : Outport  Port=2
  v_lx : Outport  Port=3
  v_ly : Outport  Port=4
  wires:
  Integrator/1 -> x_l/1, RegistroPersistente_850/1  "x_l"
  Integrator1/1 -> v_lx/1, Integrator/1, RegistroPersistente_851/1  "v_lx"
  Divide/1 -> Integrator1/1, RegistroPersistente_846/1, RegistroDisco_aceleracion_carga_x_fisica/1  "dv_lx"
  Sum/1 -> Divide/1
  F_cx/1 -> Sum/1
  Gain/1 -> Product2/1, Product/1
  F_hw/1 -> Gain/1
  theta_l/1 -> Sin2/1, Sin/1
  Sin/1 -> Product/2
  Product/1 -> Sum/2
  Divide1/1 -> Integrator3/1, RegistroPersistente_847/1, RegistroDisco_aceleracion_izaje_fisica/1  "dv_ly"
  F_cy/1 -> Sum2/3
  m_l/1 -> Divide1/2, Divide/2, Gain2/1
  Integrator3/1 -> v_ly/1, Integrator2/1, RegistroPersistente_853/1, RegistroDisco_aceleracion_carga_x_fisica_2/1  "v_ly"
  Integrator2/1 -> y_l/1, RegistroPersistente_852/1  "y_l"
  Sin2/1 -> Product2/2
  Product2/1 -> Sum2/2
  Gain2/1 -> Sum2/1
  Sum2/1 -> Divide1/1

== system Grua_MC_R2_Ciclo_Completo_SFC/Planta/Subsistema carro/Dinamica Carro Traslacional ==
  F_tw : Inport
  F_hw : Inport  Port=2
  theta_l : Inport  Port=3
  Gain : Gain  Gain=1/M_t
  Gain1 : Gain  Gain=b_t
  Gain2 : Gain  Gain=2
  Integrator : Integrator
  Integrator1 : Integrator  InitialCondition=-26.34
  Product : Product
  RegistroDisco_aceleracion_carro_fisica : Terminator
  RegistroPersistente_873 : ToWorkspace  VariableName=aceleracion_carro_fisica  SaveFormat=Timeseries  SampleTime=-1
      settings: Decimation=10
  RegistroPersistente_876 : ToWorkspace  VariableName=planta_integrador_05_Outport  SaveFormat=Timeseries  SampleTime=-1
      settings: Decimation=10
  RegistroPersistente_877 : ToWorkspace  VariableName=diag_xtrolley  SaveFormat=Timeseries  SampleTime=-1
      settings: Decimation=10
  Sin : Trigonometry
  Sum : Sum  Inputs=++-
  x_t : Outport
  v_t : Outport  Port=2
  wires:
  Sum/1 -> Gain/1
  Product/1 -> Gain2/1
  Gain/1 -> Integrator/1, RegistroPersistente_873/1, RegistroDisco_aceleracion_carro_fisica/1  "ddx_t"
  Gain2/1 -> Sum/1  "ddx_t"
  Integrator1/1 -> x_t/1, RegistroPersistente_877/1  "x_t"
  F_tw/1 -> Sum/2
  Gain1/1 -> Sum/3
  Integrator/1 -> Gain1/1, v_t/1, Integrator1/1, RegistroPersistente_876/1  "v_t"
  Sin/1 -> Product/1
  F_hw/1 -> Product/2
  theta_l/1 -> Sin/1

== system Grua_MC_R2_Ciclo_Completo_SFC/Planta/Subsistema carro/Dinamica Tambor Carro ==
  F_tw : Inport
  T_tm : Inport  Port=2
  T_tb : Inport  Port=3
  Gain3 : Gain  Gain=1/J_teq
  Gain4 : Gain  Gain=b_teq
  Gain5 : Gain  Gain=1/i_t
  Gain6 : Gain  Gain=r_td
  Gain7 : Gain  Gain=r_td
  Gain8 : Gain  Gain=r_td
  Integrator2 : Integrator
  Integrator3 : Integrator  InitialCondition=-26.34/r_td
  RegistroPersistente_888 : ToWorkspace  VariableName=planta_integrador_07_Inport  SaveFormat=Timeseries  SampleTime=-1
      settings: Decimation=10
  RegistroPersistente_892 : ToWorkspace  VariableName=diag_xdrum  SaveFormat=Timeseries  SampleTime=-1
      settings: Decimation=10
  RegistroPersistente_893 : ToWorkspace  VariableName=diag_vdrum  SaveFormat=Timeseries  SampleTime=-1
      settings: Decimation=10
  RegistroPersistente_894 : ToWorkspace  VariableName=planta_integrador_07_Outport  SaveFormat=Timeseries  SampleTime=-1
      settings: Decimation=10
  RegistroPersistente_895 : ToWorkspace  VariableName=planta_integrador_08_Outport  SaveFormat=Timeseries  SampleTime=-1
      settings: Decimation=10
  Sum1 : Sum  Inputs=++--
  x_td : Outport
  dx_td : Outport  Port=2
  theta_td : Outport  Port=3
  omega_td : Outport  Port=4
  wires:
  Gain3/1 -> Integrator2/1, RegistroPersistente_888/1  "ddtheta_td"
  Integrator2/1 -> omega_td/1, Gain4/1, Gain8/1, Integrator3/1, RegistroPersistente_894/1  "omega_td"
  Sum1/1 -> Gain3/1
  T_tb/1 -> Sum1/2
  Integrator3/1 -> Gain7/1, theta_td/1, RegistroPersistente_895/1  "theta_td"
  Gain6/1 -> Gain5/1  "T_tdl"
  Gain4/1 -> Sum1/4
  Gain5/1 -> Sum1/3  "ddtheta_td"
  T_tm/1 -> Sum1/1
  Gain7/1 -> x_td/1, RegistroPersistente_892/1  "x_td"
  Gain8/1 -> dx_td/1, RegistroPersistente_893/1  "dx_td"
  F_tw/1 -> Gain6/1

== system Grua_MC_R2_Ciclo_Completo_SFC/Planta/Subsistema carro/Dinamica cable carro ==
  x_t : Inport
  dx_t : Inport  Port=2
  x_td : Inport  Port=3
  dx_td : Inport  Port=4
  Gain10 : Gain  Gain=b_tw
  Gain9 : Gain  Gain=K_tw
  Sum2 : Sum  Inputs=|+-
  Sum3 : Sum  Inputs=|+-
  Sum4 : Sum
  F_tw : Outport
  wires:
  x_t/1 -> Sum2/2
  Gain9/1 -> Sum4/1  "T_tdl"
  Sum4/1 -> F_tw/1  "F_tw"
  dx_t/1 -> Sum3/2
  dx_td/1 -> Sum3/1
  Sum2/1 -> Gain9/1
  Sum3/1 -> Gain10/1
  x_td/1 -> Sum2/1
  Gain10/1 -> Sum4/2  "T_tdl"

== system Grua_MC_R2_Ciclo_Completo_SFC/Planta/Subsistema carro/Modelo Freno Operacion Carro ==
  BRK_t : Inport
  omega_tm : Inport  Port=2
  Constant : Constant  Value=0
  Gain : Gain  Gain=-b_tb
  RegistroPersistente_915 : ToWorkspace  VariableName=diag_brake_torque  SaveFormat=Timeseries  SampleTime=-1
      settings: Decimation=10
  Saturation : Saturate  UpperLimit=T_tbMax  LowerLimit=-T_tbMax
  Switch : Switch  Criteria=u2 > Threshold  SaturateOnIntegerOverflow=off  InputSameDT=off
  T_tb : Outport
  wires:
  Saturation/1 -> Switch/3
  omega_tm/1 -> Gain/1
  Switch/1 -> T_tb/1, RegistroPersistente_915/1
  Gain/1 -> Saturation/1
  Constant/1 -> Switch/1
  BRK_t/1 -> Switch/2

== system Grua_MC_R2_Ciclo_Completo_SFC/Planta/Subsistema carro/Modulador de Torque Motor Drive Carro ==
  T_tm* : Inport
  Diferencia torque saturacion : Sum  Inputs=+-
  Gain : Gain  Gain=1/tau_tm
  Integrator : Integrator
  RegistroPersistente_919 : ToWorkspace  VariableName=aw_delta_torque_Nm  SaveFormat=Timeseries  SampleTime=-1
      settings: Decimation=10
  RegistroPersistente_920 : ToWorkspace  VariableName=planta_integrador_09_Inport  SaveFormat=Timeseries  SampleTime=-1
      settings: Decimation=10
  RegistroPersistente_921 : ToWorkspace  VariableName=planta_integrador_09_Outport  SaveFormat=Timeseries  SampleTime=-1
      settings: Decimation=10
  RegistroPersistente_922 : ToWorkspace  VariableName=T_tmlim_  SaveFormat=Timeseries  SampleTime=-1
      settings: Decimation=10
  Saturation : Saturate  UpperLimit=T_tmMax  LowerLimit=-T_tmMax
  Sum : Sum  Inputs=|+-
  T_tm : Outport
  Delta torque limite : Outport  Port=2
  wires:
  Integrator/1 -> Sum/2, T_tm/1, RegistroPersistente_921/1
  Gain/1 -> Integrator/1, RegistroPersistente_920/1
  Sum/1 -> Gain/1
  Saturation/1 -> Sum/1, Diferencia torque saturacion/1, RegistroPersistente_922/1  "T_tmlim*"
  T_tm*/1 -> Saturation/1, Diferencia torque saturacion/2
  Diferencia torque saturacion/1 -> Delta torque limite/1, RegistroPersistente_919/1

== system Grua_MC_R2_Ciclo_Completo_SFC/Planta/Subsistema izaje/Calculo longitud l_h ==
  note: $\dot{l}_h(t)=-\frac{r_{hd}}{2}\omega_{hd}(t)$
  omega_hd : Inport
  Gain : Gain  Gain=-r_hd/2
  Integrator : Integrator  InitialCondition=l_hi
  RegistroPersistente_937 : ToWorkspace  VariableName=planta_integrador_10_Inport  SaveFormat=Timeseries  SampleTime=-1
      settings: Decimation=10
  RegistroPersistente_938 : ToWorkspace  VariableName=planta_integrador_10_Outport  SaveFormat=Timeseries  SampleTime=-1
      settings: Decimation=10
  l_h : Outport
  dl_h : Outport  Port=2
  wires:
  Integrator/1 -> l_h/1, RegistroPersistente_938/1  "l_h"
  omega_hd/1 -> Gain/1
  Gain/1 -> dl_h/1, Integrator/1, RegistroPersistente_937/1  "dl_h"

== system Grua_MC_R2_Ciclo_Completo_SFC/Planta/Subsistema izaje/Dinamica Tambor Izaje ==
  T_hEb : Inport
  T_hm : Inport  Port=2
  F_hw : Inport  Port=3
  T_hb : Inport  Port=4
  Gain1 : Gain  Gain=r_hd
  Gain2 : Gain  Gain=1/i_h
  Gain3 : Gain  Gain=1/J_heq
  Gain4 : Gain  Gain=b_heq
  Gain5 : Gain  Gain=1/i_h
  Integrator2 : Integrator
  Integrator3 : Integrator
  RegistroPersistente_947 : ToWorkspace  VariableName=planta_integrador_11_Inport  SaveFormat=Timeseries  SampleTime=-1
      settings: Decimation=10
  RegistroPersistente_950 : ToWorkspace  VariableName=planta_integrador_11_Outport  SaveFormat=Timeseries  SampleTime=-1
      settings: Decimation=10
  RegistroPersistente_951 : ToWorkspace  VariableName=planta_integrador_12_Outport  SaveFormat=Timeseries  SampleTime=-1
      settings: Decimation=10
  Sum1 : Sum  Inputs=+++--
  theta_hd : Outport
  omega_hd : Outport  Port=2
  wires:
  Gain3/1 -> Integrator2/1, RegistroPersistente_947/1  "ddtheta_hd"
  Integrator2/1 -> omega_hd/1, Gain4/1, Integrator3/1, RegistroPersistente_950/1  "omega_hd"
  Sum1/1 -> Gain3/1
  T_hb/1 -> Sum1/2
  T_hEb/1 -> Gain5/1  "T_hEb"
  Gain4/1 -> Sum1/5
  Gain5/1 -> Sum1/3
  T_hm/1 -> Sum1/1
  F_hw/1 -> Gain1/1
  Gain1/1 -> Gain2/1  "T_hdl"
  Gain2/1 -> Sum1/4
  Integrator3/1 -> theta_hd/1, RegistroPersistente_951/1  "theta_hd"

== system Grua_MC_R2_Ciclo_Completo_SFC/Planta/Subsistema izaje/Dinamica cable Izaje ==
  note: b_hw
  note: K_hw
  l : Inport
  l_h : Inport  Port=2
  dl : Inport  Port=3
  dl_h : Inport  Port=4
  Constant : Constant  Value=0
  Constant1 : Constant  Value=k_wu
  Constant2 : Constant  Value=L_h0
  Constant3 : Constant  Value=L_h0
  Divide : Product  Inputs=*/
  Gain{,1..2,4} (4 alike) : Gain  Gain=2
  Gain3 : Gain  Gain=b_wu
  Product : Product
  Product1 : Product
  Sum : Sum  Inputs=+-
  Sum1 : Sum
  Sum2 : Sum  Inputs=+-
  Sum3 : Sum
  Sum4 : Sum  Inputs=|++
  Switch : Switch  SaturateOnIntegerOverflow=off  InputSameDT=off
  F_hw : Outport
  wires:
  Constant/1 -> Switch/3
  l/1 -> Sum/1
  l_h/1 -> Gain4/1, Sum/2, Gain/1  "l_h"
  Sum/1 -> Switch/2, Gain1/1
  Switch/1 -> F_hw/1
  Sum1/1 -> Switch/1
  Gain1/1 -> Product/2
  Product/1 -> Sum1/1
  Divide/1 -> Product/1  "K_hw"
  Gain3/1 -> Product1/2  "b_hw"
  dl/1 -> Sum2/1  "dl"
  dl_h/1 -> Sum2/2  "dl_h"
  Sum2/1 -> Gain2/1
  Gain2/1 -> Product1/1
  Product1/1 -> Sum1/2
  Sum3/1 -> Divide/2
  Constant1/1 -> Divide/1
  Constant2/1 -> Sum3/2
  Gain/1 -> Sum3/1
  Gain4/1 -> Sum4/1
  Sum4/1 -> Gain3/1
  Constant3/1 -> Sum4/2

== system Grua_MC_R2_Ciclo_Completo_SFC/Planta/Subsistema izaje/Modelo Freno Emergencia de Izaje(Eje lento) ==
  omega_hd : Inport
  BRK_hE : Inport  Port=2
  Constant : Constant  Value=0
  Gain : Gain  Gain=-b_hEb
  Saturation : Saturate  UpperLimit=T_hEbMax  LowerLimit=-T_hEbMax
  Switch : Switch  Criteria=u2 > Threshold  SaturateOnIntegerOverflow=off  InputSameDT=off
  T_hEb : Outport
  wires:
  Saturation/1 -> Switch/3
  omega_hd/1 -> Gain/1
  Switch/1 -> T_hEb/1
  Gain/1 -> Saturation/1
  Constant/1 -> Switch/1
  BRK_hE/1 -> Switch/2

== system Grua_MC_R2_Ciclo_Completo_SFC/Planta/Subsistema izaje/Modelo Freno Operacion de Izaje(Eje Rapido) ==
  BRK_h : Inport
  omega_hm : Inport  Port=2
  Constant : Constant  Value=0
  Gain : Gain  Gain=-b_hb
  Saturation : Saturate  UpperLimit=T_hbMax  LowerLimit=-T_hbMax
  Switch : Switch  Criteria=u2 > Threshold  SaturateOnIntegerOverflow=off  InputSameDT=off
  T_hb : Outport
  wires:
  Saturation/1 -> Switch/3
  omega_hm/1 -> Gain/1
  Switch/1 -> T_hb/1
  Gain/1 -> Saturation/1
  Constant/1 -> Switch/1
  BRK_h/1 -> Switch/2

== system Grua_MC_R2_Ciclo_Completo_SFC/Planta/Subsistema izaje/Modulador de Torque Motor Drive Izaje ==
  T_hm* : Inport
  omega_hm : Inport  Port=2
  Calculo Torque Limite : Subsystem
  Gain : Gain  Gain=1/tau_hm
  Gain1 : Gain  Gain=-1
  Integrator : Integrator
  RegistroPersistente_1005 : ToWorkspace  VariableName=planta_integrador_13_Inport  SaveFormat=Timeseries  SampleTime=-1
      settings: Decimation=10
  RegistroPersistente_1007 : ToWorkspace  VariableName=planta_integrador_13_Outport  SaveFormat=Timeseries  SampleTime=-1
      settings: Decimation=10
  RegistroPersistente_1008 : ToWorkspace  VariableName=Thm_sat  SaveFormat=Timeseries  SampleTime=-1
      settings: Decimation=10
  Saturation Dynamic : simulink/Discontinuities/Saturation Dynamic  OutMin=[]  OutMax=[]  OutDataTypeStr=Inherit: Same as second input  OutDataType=fixdt(1, 16)  OutScaling=2^-10  DoSatur=off
  Sum : Sum  Inputs=|+-
  T_hm : Outport
  wires:
  Gain/1 -> Integrator/1, RegistroPersistente_1005/1
  Sum/1 -> Gain/1
  Integrator/1 -> T_hm/1, Sum/2, RegistroPersistente_1007/1
  Saturation Dynamic/1 -> Sum/1, RegistroPersistente_1008/1  "Thm_sat"
  T_hm*/1 -> Saturation Dynamic/2
  omega_hm/1 -> Calculo Torque Limite/1(omega_hm)
  Calculo Torque Limite/1(T_hmMax) -> Gain1/1, Saturation Dynamic/1
  Gain1/1 -> Saturation Dynamic/3

== system Grua_MC_R2_Ciclo_Completo_SFC/Planta/Subsistema izaje/Modulador de Torque Motor Drive Izaje/Calculo Torque Limite ==
  omega_hm : Inport
  Abs omega : Abs  SaturateOnIntegerOverflow=off
  Constant2 : Constant
  Divide : Product  Inputs=*/
  Gain1 : Gain  Gain=T_hmMax
  Min : MinMax  Inputs=2
  Proteccion omega cero : Saturate  UpperLimit=inf  LowerLimit=1e-6
  RegistroPersistente_1000 : ToWorkspace  VariableName=T_hmMax  SaveFormat=Timeseries  SampleTime=-1
      settings: Decimation=10
  Square : Math  Operator=square
  omega_hmRATED : Constant  Value=omega_hmRATED
  T_hmMax : Outport
  wires:
  omega_hmRATED/1 -> Divide/1
  Gain1/1 -> T_hmMax/1, RegistroPersistente_1000/1  "T_hmMax"
  Min/1 -> Gain1/1
  Constant2/1 -> Min/2
  Square/1 -> Min/1
  Divide/1 -> Square/1
  omega_hm/1 -> Abs omega/1
  Abs omega/1 -> Proteccion omega cero/1
  Proteccion omega cero/1 -> Divide/2

== stateflow chart Grua_MC_R2_Ciclo_Completo_SFC/PICK // PLACE ==
  state INICIO
    entry:
    evento_cambio = false;
    tipo_evento = 0;
    slot_evento = -1;
    slot_mem = -1;
    carga_tomada = TLK;
  state VACIO1
    during:
    evento_cambio = false;
    tipo_evento = 0;
    slot_evento = -1;
    carga_tomada = 0;
  state PRE_PLACE
    during:
    evento_cambio = false;
    tipo_evento = 0;
    slot_evento = -1;
    carga_tomada = 1;
  state CARGADO1
    during:
    evento_cambio = false;
    tipo_evento = 0;
    slot_evento = -1;
    carga_tomada = 1;
  state PRE_PICK
    during:
    evento_cambio = false;
    tipo_evento = 0;
    slot_evento = -1;
    carga_tomada = 0;
  (default) -> ? [commented out]
  (default) -> ? [commented out] : [slot_ok && TLK == 1 && tension && ~contacto && v_yl > -0.05]{slot_evento = k_slot;}
  (default) -> ? [commented out] : [slot_ok && TLK == 0 && ~tension && contacto && abs(v_yl) < 0.05]{slot_evento = k_slot;}
  (default) -> ? [commented out] : [true]
  (default) -> INICIO
  INICIO -> VACIO1 [order 1] : [TLK==0]
  INICIO -> CARGADO1 [order 2] : [TLK ==1]
  PRE_PLACE -> VACIO1 [order 2] : [slot_ok && TLK == 0 && contacto]{evento_cambio = true; tipo_evento = 2; slot_evento = slot_mem;}
  CARGADO1 -> PRE_PLACE : [slot_ok && TLK == 1 && contacto && abs(v_yl) < 0.05]{slot_mem = k_slot;}
  PRE_PICK -> VACIO1 [order 1] : [~slot_ok || (~contacto && TLK == 0)]{slot_mem = -1;}
  PRE_PLACE -> CARGADO1 [order 1] : [TLK == 1 && tension && ~contacto && v_yl > 0.05]{slot_mem = -1;}
  VACIO1 -> PRE_PICK : [slot_ok && contacto && TLK == 0]{slot_mem = k_slot;}
  PRE_PICK -> CARGADO1 [order 2] : [slot_ok && TLK == 1 && tension && ~contacto && v_yl > 0.05]{evento_cambio = true; tipo_evento = 1; slot_evento = slot_mem;}
  data: TLK input; k_slot input; slot_ok input; v_yl input; evento_cambio output; tipo_evento output; slot_evento output int32; contacto input; tension input; slot_mem local int32; carga_tomada output

== matlab function Grua_MC_R2_Ciclo_Completo_SFC/Histeresis_F_hw ==
  data: F_hw input; tension output
function tension = tension_hist_Fhw(F_hw)
% Histeresis física para detectar "cable cargado" a partir de F_hw [N].
% Basada en fracciones del peso mínimo (spreader + contenedor vacío).

% --- Parámetros físicos ---
g = 9.81;
M_s    = 15000;   % kg
M_cmin = 2000;    % kg

Wmin = (M_s + M_cmin) * g;     % N  ~ 167 kN

% --- Umbrales con histéresis ---
Fhw_on  = 0.21 * Wmin;         % ~ 35 kN (cable claramente cargado)
Fhw_off = 0.09 * Wmin;         % ~ 15 kN (cable claramente descargado)

% --- Estado persistente ---
persistent t
if isempty(t)
    t = false;
end

% --- Lógica de histéresis ---
if ~t
    if F_hw > Fhw_on
        t = true;
    end
else
    if F_hw < Fhw_off
        t = false;
    end
end

tension = t;
end
